simulink model "Design_5new_300000"  (R2026a)
settings: Solver=FixedStepAuto  StopTime=300000  FixedStep=300
undefined symbols (not defined in the file): coloring, m, n, tamk, vapor
libraries: mqttlib x7
(part 2 of 2)

== matlab function Design_5new_300000/MATLAB Function ==
  data: d input; payload output double size=1


%function payload = fcn(d)
%#codegen

%payload = double(d);

%end


%function payload = fcn(d)
%#codegen

%payload = 1.0;
%payload = uint8(1);
%payload = uint8('1');
%payload = uint8(49);   % ASCII '1'
%payload = '1';

%end

%%

function payload = fcn(d)
%#codegen

if d > 0
    payload = 1.0;   % Blasting completed
else
    payload = 0.0;
end

end

== matlab function Design_5new_300000/MATLAB Function1 ==
  data: d input; payload output double size=1



%function payload = fcn(d)
%#codegen

%payload = double(d);

%end

%%

%function payload = fcn(d)

%#codegen

%payload = 3.0;
%payload = uint8(3);
%payload = uint8('3');
%payload = uint8(51);   % ASCII '3'
%payload = '3';

%end


%%

function payload = fcn(d)
%#codegen

if d > 0
    payload = 3.0;   % Surfacing completed
else
    payload = 0.0;
end

end

== matlab function Design_5new_300000/MATLAB Function2 ==
  data: d input; payload output double size=1


%function payload = fcn(d)
%#codegen

%payload = double(d);

%end

%%

%function payload = fcn(d)
%#codegen

%payload = 4.0;
%payload = uint8(4);
%payload = uint8('4');
%payload = uint8(52);   % '4'
%payload = '4';


%end


%%

function payload = fcn(d)
%#codegen

if d > 0
    payload = 4.0;   % Coloring completed
else
    payload = 0.0;
end

end

== matlab function Design_5new_300000/MATLAB Function3 ==
  data: d input; payload output double size=1

%function payload = fcn(d)


%function payload = fcn(d)
%#codegen

%if d > 0
  % payload = uint8(53);   % ASCII '5' = Vapor completed
%else
    %payload = uint8(48);   % ASCII '0' = no vapor yet
%end

%end

%%
%function payload = fcn(d)
%#codegen

%if d > 0
    %payload = 5.0;   % Vapor completed
%else
    %payload = 0.0;   % No vapor event
%end

%end

%%

function payload = fcn(d)
%#codegen

if d > 0
    payload = 5.0;   % Vapor completed
else
    payload = 0.0;
end

end
